simulink model "identificamodels"  (R2017b)
settings: Solver=ode4  StartTime=0.0  StopTime=75  FixedStep=1e-3  RelTol=1e-3
values from neighbouring files (symbols this model uses):
  dGz = [1,zeros(1,length(yk)-1)]    [ssoidentifica.m]
  KP = TI/(0.5*(2*b+td))    (= 0.356749812536)    [ssoidentifica.m]
  nGz = hk'    [ssoidentifica.m]
  TD = TI-2*xi*tau+tau^2/TI-td^3/(6*TI*(2*b+td))    (= 8.8094809298)    [ssoidentifica.m]
  TI = 2*xi*tau-(2*b^2-td^2)/(2*(2*b+td))    (= 0.428099775043)    [ssoidentifica.m]
  Tm = 1    [ssoidentifica.m]
settings Model: Creator=pablo  LastModifiedBy=pablo

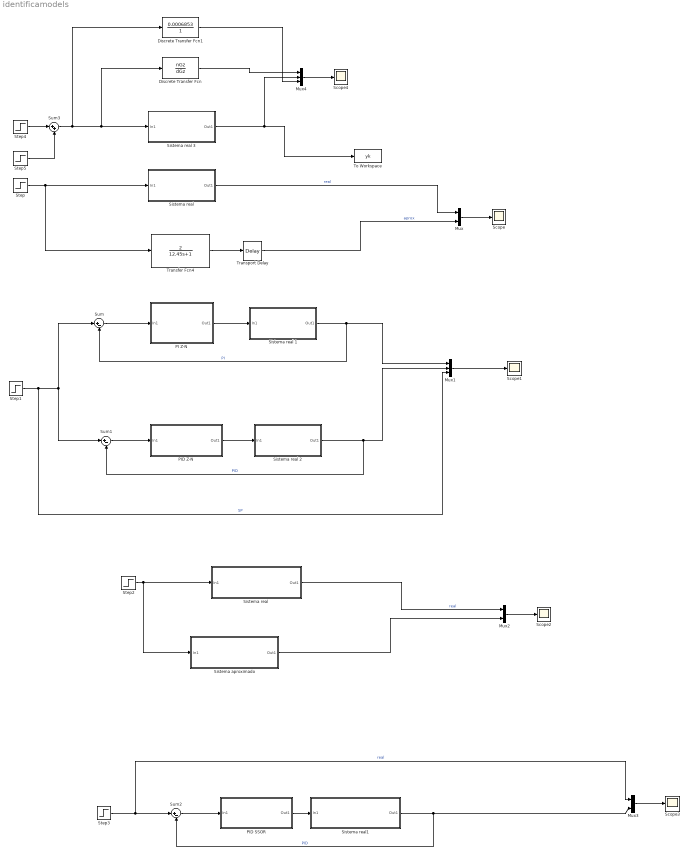
== system identificamodels ==
  Discrete Transfer Fcn : DiscreteTransferFcn  Numerator=nGz  Denominator=dGz  SampleTime=Tm
  Discrete Transfer Fcn1 : DiscreteTransferFcn  Numerator=[0.0006853]  Denominator=[1]  SampleTime=Tm
  Mux : Mux  Inputs=2
  Mux1 : Mux  Inputs=3
  Mux2 : Mux  Inputs=2
  Mux3 : Mux  Inputs=2
  Mux4 : Mux  Inputs=3
  "PI Z-N " : Subsystem
  "PID SSOR " : Subsystem
  "PID Z-N " : Subsystem
  Scope{,1..4} (5 alike) : Scope
  "Sistema aproximado " : Subsystem
  Sistema real : Subsystem
  "Sistema real " : Subsystem
  Sistema real 1 : Subsystem
  Sistema real 2 : Subsystem
  Sistema real 3 : Subsystem
  Sistema real1 : Subsystem
  Step : Step  Time=0  After=0.5  SampleTime=0
  Step1 : Step  Time=0  After=0.4  SampleTime=0
  Step2 : Step  Time=0  SampleTime=0
  Step3 : Step  Time=0  SampleTime=0
  Step4 : Step  Time=0  After=0.5  SampleTime=0
  Step5 : Step  After=-0.5  SampleTime=0
  Sum : Sum  Inputs=|+-
  Sum1 : Sum  Inputs=|+-
  Sum2 : Sum  Inputs=|+-
  Sum3 : Sum  Inputs=|++
  To Workspace : ToWorkspace  VariableName=yk  SampleTime=-1
      settings: Decimation=1e3
  Transfer Fcn4 : TransferFcn  Numerator=[2]  Denominator=[12.45 1]
  Transport Delay : TransportDelay  DelayTime=6.4
  wires:
  Step/1 -> Transfer Fcn4/1, "Sistema real "/1(In1)
  Transfer Fcn4/1 -> Transport Delay/1
  "PI Z-N "/1(Out1) -> Sistema real 1/1(In1)
  Mux/1 -> Scope/1
  Transport Delay/1 -> Mux/2  "aprox"
  "Sistema real "/1(Out1) -> Mux/1  "real"
  Sum/1 -> "PI Z-N "/1(In1)
  Sistema real 1/1(Out1) -> Sum/2, Mux1/1  "PI"
  Sistema real 2/1(Out1) -> Sum1/2, Mux1/2  "PID"
  Mux1/1 -> Scope1/1
  "PID Z-N "/1(Out1) -> Sistema real 2/1(In1)
  Sum1/1 -> "PID Z-N "/1(In1)
  Step1/1 -> Mux1/3, Sum1/1, Sum/1  "SP"
  Step2/1 -> "Sistema aproximado "/1(In1), Sistema real/1(In1)
  Sistema real/1(Out1) -> Mux2/1  "real"
  Mux2/1 -> Scope2/1
  "Sistema aproximado "/1(Out1) -> Mux2/2
  Sum2/1 -> "PID SSOR "/1(In1)
  "PID SSOR "/1(Out1) -> Sistema real1/1(In1)
  Sistema real1/1(Out1) -> Sum2/2, Mux3/2  "PID"
  Mux3/1 -> Scope3/1
  Step3/1 -> Mux3/1, Sum2/1  "real"
  Step4/1 -> Sum3/1
  Step5/1 -> Sum3/2
  Sum3/1 -> Discrete Transfer Fcn1/1, Discrete Transfer Fcn/1, Sistema real 3/1(In1)
  Sistema real 3/1(Out1) -> Mux4/2, To Workspace/1
  Mux4/1 -> Scope4/1
  Discrete Transfer Fcn/1 -> Mux4/1
  Discrete Transfer Fcn1/1 -> Mux4/3

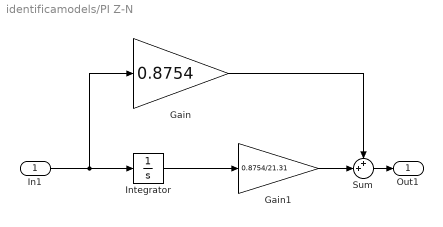
== system identificamodels/PI Z-N  ==
  In1 : Inport
  Gain : Gain  Gain=0.8754
  Gain1 : Gain  Gain=0.8754/21.31
  Integrator : Integrator
  Sum : Sum  Inputs=++|
  Out1 : Outport
  wires:
  Gain/1 -> Sum/1
  Gain1/1 -> Sum/2
  Integrator/1 -> Gain1/1
  Sum/1 -> Out1/1
  In1/1 -> Gain/1, Integrator/1

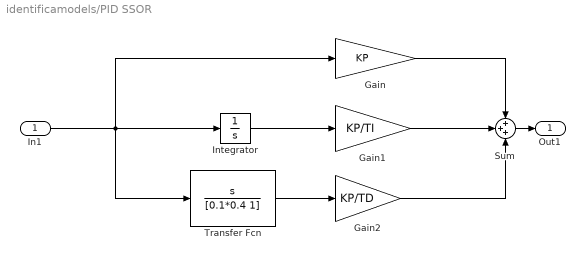
== system identificamodels/PID SSOR  ==
  In1 : Inport
  Gain : Gain  Gain=KP
  Gain1 : Gain  Gain=KP/TI
  Gain2 : Gain  Gain=KP/TD
  Integrator : Integrator
  Sum : Sum  Inputs=+++
  Transfer Fcn : TransferFcn  Numerator=[1 0]  Denominator=[0.1*0.4 1]
  Out1 : Outport
  wires:
  Gain/1 -> Sum/1
  Integrator/1 -> Gain1/1
  Gain2/1 -> Sum/3
  In1/1 -> Gain/1, Transfer Fcn/1, Integrator/1
  Gain1/1 -> Sum/2
  Sum/1 -> Out1/1
  Transfer Fcn/1 -> Gain2/1

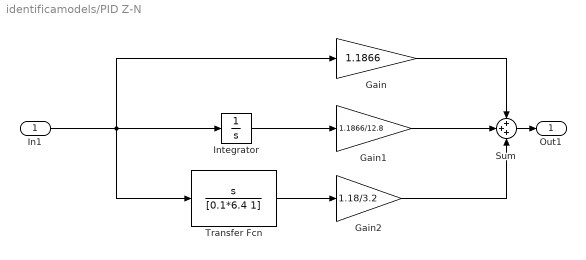
== system identificamodels/PID Z-N  ==
  In1 : Inport
  Gain : Gain  Gain=1.1866
  Gain1 : Gain  Gain=1.1866/12.8
  Gain2 : Gain  Gain=1.18/3.2
  Integrator : Integrator
  Sum : Sum  Inputs=+++
  Transfer Fcn : TransferFcn  Numerator=[1 0]  Denominator=[0.1*6.4 1]
  Out1 : Outport
  wires:
  Gain/1 -> Sum/1
  Integrator/1 -> Gain1/1
  Gain2/1 -> Sum/3
  In1/1 -> Gain/1, Transfer Fcn/1, Integrator/1
  Gain1/1 -> Sum/2
  Sum/1 -> Out1/1
  Transfer Fcn/1 -> Gain2/1

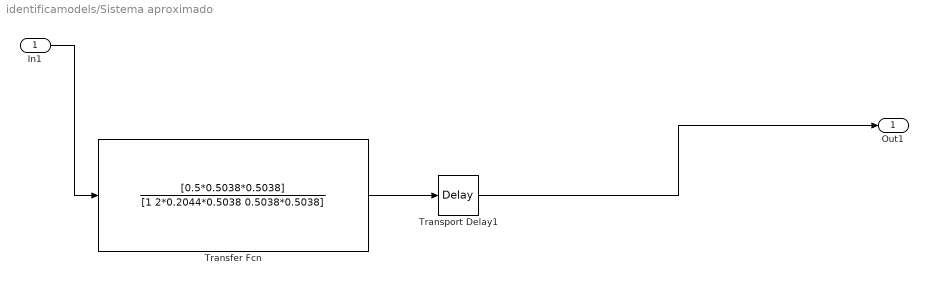
== system identificamodels/Sistema aproximado  ==
  In1 : Inport
  Transfer Fcn : TransferFcn  Numerator=[0.5*0.5038*0.5038]  Denominator=[1 2*0.2044*0.5038 0.5038*0.5038]
  Transport Delay1 : TransportDelay  DelayTime=0.4
  Out1 : Outport
  wires:
  Transport Delay1/1 -> Out1/1
  In1/1 -> Transfer Fcn/1
  Transfer Fcn/1 -> Transport Delay1/1

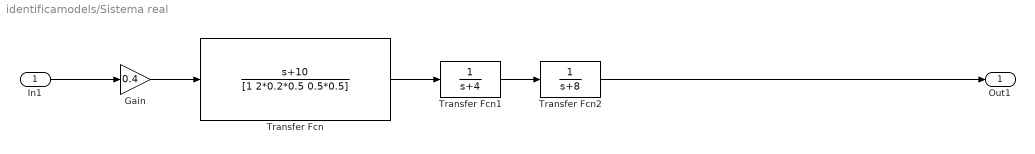
== system identificamodels/Sistema real ==
  In1 : Inport
  Gain : Gain  Gain=0.4
  Transfer Fcn : TransferFcn  Numerator=[1 10]  Denominator=[1 2*0.2*0.5 0.5*0.5]
  Transfer Fcn1 : TransferFcn  Denominator=[1 4]
  Transfer Fcn2 : TransferFcn  Denominator=[1 8]
  Out1 : Outport
  wires:
  In1/1 -> Gain/1
  Transfer Fcn/1 -> Transfer Fcn1/1
  Gain/1 -> Transfer Fcn/1
  Transfer Fcn1/1 -> Transfer Fcn2/1
  Transfer Fcn2/1 -> Out1/1

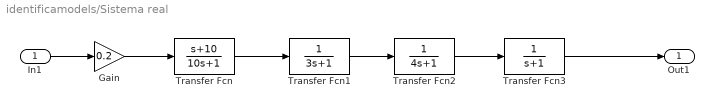
== system identificamodels/Sistema real  ==
  In1 : Inport
  Gain : Gain  Gain=0.2
  Transfer Fcn : TransferFcn  Numerator=[1 10]  Denominator=[10 1]
  Transfer Fcn1 : TransferFcn  Denominator=[3 1]
  Transfer Fcn2 : TransferFcn  Denominator=[4 1]
  Transfer Fcn3 : TransferFcn  Denominator=[1 1]
  Out1 : Outport
  wires:
  In1/1 -> Gain/1
  Transfer Fcn2/1 -> Transfer Fcn3/1
  Transfer Fcn/1 -> Transfer Fcn1/1
  Transfer Fcn1/1 -> Transfer Fcn2/1
  Gain/1 -> Transfer Fcn/1
  Transfer Fcn3/1 -> Out1/1

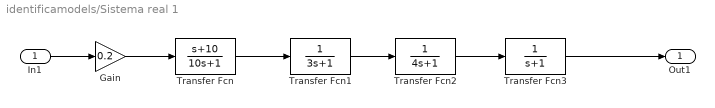
== system identificamodels/Sistema real 1 ==
  In1 : Inport
  Gain : Gain  Gain=0.2
  Transfer Fcn : TransferFcn  Numerator=[1 10]  Denominator=[10 1]
  Transfer Fcn1 : TransferFcn  Denominator=[3 1]
  Transfer Fcn2 : TransferFcn  Denominator=[4 1]
  Transfer Fcn3 : TransferFcn  Denominator=[1 1]
  Out1 : Outport
  wires:
  In1/1 -> Gain/1
  Transfer Fcn2/1 -> Transfer Fcn3/1
  Transfer Fcn/1 -> Transfer Fcn1/1
  Transfer Fcn1/1 -> Transfer Fcn2/1
  Gain/1 -> Transfer Fcn/1
  Transfer Fcn3/1 -> Out1/1

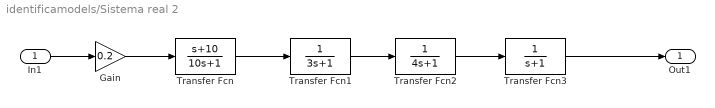
== system identificamodels/Sistema real 2 ==
  In1 : Inport
  Gain : Gain  Gain=0.2
  Transfer Fcn : TransferFcn  Numerator=[1 10]  Denominator=[10 1]
  Transfer Fcn1 : TransferFcn  Denominator=[3 1]
  Transfer Fcn2 : TransferFcn  Denominator=[4 1]
  Transfer Fcn3 : TransferFcn  Denominator=[1 1]
  Out1 : Outport
  wires:
  In1/1 -> Gain/1
  Transfer Fcn2/1 -> Transfer Fcn3/1
  Transfer Fcn/1 -> Transfer Fcn1/1
  Transfer Fcn1/1 -> Transfer Fcn2/1
  Gain/1 -> Transfer Fcn/1
  Transfer Fcn3/1 -> Out1/1

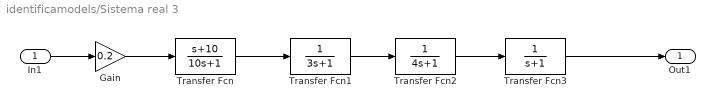
== system identificamodels/Sistema real 3 ==
  In1 : Inport
  Gain : Gain  Gain=0.2
  Transfer Fcn : TransferFcn  Numerator=[1 10]  Denominator=[10 1]
  Transfer Fcn1 : TransferFcn  Denominator=[3 1]
  Transfer Fcn2 : TransferFcn  Denominator=[4 1]
  Transfer Fcn3 : TransferFcn  Denominator=[1 1]
  Out1 : Outport
  wires:
  In1/1 -> Gain/1
  Transfer Fcn2/1 -> Transfer Fcn3/1
  Transfer Fcn/1 -> Transfer Fcn1/1
  Transfer Fcn1/1 -> Transfer Fcn2/1
  Gain/1 -> Transfer Fcn/1
  Transfer Fcn3/1 -> Out1/1

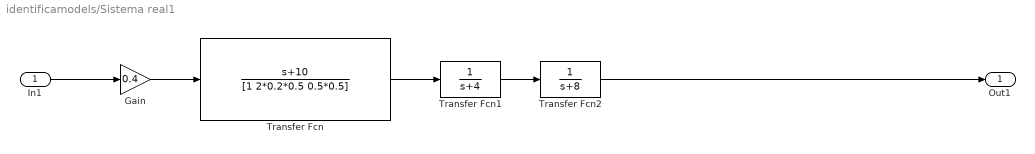
== system identificamodels/Sistema real1 ==
  In1 : Inport
  Gain : Gain  Gain=0.4
  Transfer Fcn : TransferFcn  Numerator=[1 10]  Denominator=[1 2*0.2*0.5 0.5*0.5]
  Transfer Fcn1 : TransferFcn  Denominator=[1 4]
  Transfer Fcn2 : TransferFcn  Denominator=[1 8]
  Out1 : Outport
  wires:
  In1/1 -> Gain/1
  Transfer Fcn/1 -> Transfer Fcn1/1
  Gain/1 -> Transfer Fcn/1
  Transfer Fcn1/1 -> Transfer Fcn2/1
  Transfer Fcn2/1 -> Out1/1
